simulink model "VehCtrlMdel240912_2018b"  (R2019b)
settings: Solver=FixedStepDiscrete  StartTime=0.0  StopTime=10.0  FixedStep=0.0005  RelTol=1e-3  EnableMultiTasking=on
values from neighbouring files (symbols this model uses):
  Ax_OffSet = 0.0    [VehCtrlMdelDictionary.sldd]
  Ay_OffSet = 0.0    [VehCtrlMdelDictionary.sldd]
  Caf = 460.0    [VehCtrlMdelDictionary.sldd]    (also in trqvparameter.m = 460)
  Car = 440.0    [VehCtrlMdelDictionary.sldd]    (also in trqvparameter.m = 440)
  dwf = 1.2    [VehCtrlMdelDictionary.sldd]    (also in trqvparameter.m)
  dwr = 1.2    [VehCtrlMdelDictionary.sldd]    (also in trqvparameter.m)
  h = 0.29    [VehCtrlMdelDictionary.sldd]    (also in trqvparameter.m)
  i1 = 11.4    [VehCtrlMdelDictionary.sldd]    (also in trqvparameter.m)
  i2 = 3.4    [VehCtrlMdelDictionary.sldd]    (also in trqvparameter.m)
  Iz = 105.0    [VehCtrlMdelDictionary.sldd]    (also in trqvparameter.m = 105)
  Kc = 1.0    [VehCtrlMdelDictionary.sldd]    (also in trqvparameter.m = 1)
  Ki = 1.0    [VehCtrlMdelDictionary.sldd]    (also in trqvparameter.m = 5)
  Ldwf = 1.2    [VehCtrlMdelDictionary.sldd]    (also in trqvparameter.m)
  Ldwr = 1.16    [VehCtrlMdelDictionary.sldd]    (also in trqvparameter.m)
  lf = 0.761    [VehCtrlMdelDictionary.sldd]    (also in trqvparameter.m)
  lr = 0.831    [VehCtrlMdelDictionary.sldd]    (also in trqvparameter.m)
  m = 340.0    [VehCtrlMdelDictionary.sldd]    (also in trqvparameter.m = 340)
  Offset_Angle = 0.0    [VehCtrlMdelDictionary.sldd]
  Qa = 0.1    [VehCtrlMdelDictionary.sldd]    (also in trqvparameter.m)
  Ra = 2.0    [VehCtrlMdelDictionary.sldd]    (also in trqvparameter.m = 2)
  Rt = 0.2    [VehCtrlMdelDictionary.sldd]    (also in trqvparameter.m)
  thr1 = 2.0    [VehCtrlMdelDictionary.sldd]    (also in trqvparameter.m = 2)
  thr2 = 0.5    [VehCtrlMdelDictionary.sldd]    (also in trqvparameter.m)
  thr3 = 0.8    [VehCtrlMdelDictionary.sldd]    (also in trqvparameter.m)
  thr4 = 0.5    [VehCtrlMdelDictionary.sldd]    (also in trqvparameter.m)
  thr5 = -0.5    [VehCtrlMdelDictionary.sldd]    (also in trqvparameter.m)
  TrqRquRate = 0.1    [VehCtrlMdelDictionary.sldd]    (also in trqvparameter.m)
  YawRate_OffSet = 0.0    [VehCtrlMdelDictionary.sldd]
undefined symbols (not defined in the file or in its folder): DiscIntNeverNeededParam, I_AN07_5V, I_AN08_5V, I_AN10_5V, I_SW01_L, I_SW02_L, I_SW03_L, O_SW12_HS1A, O_SW14_HS1A, PWM3
libraries: simulink x141, ec5744lib x77, canmsglib x18
(part 1 of 5)
settings Model: DataDictionary=VehCtrlMdelDictionary.sldd  EnableAccessToBaseWorkspace=off  Creator=YJR  LastModifiedBy=12045
settings DataIOCC: ReturnWorkspaceOutputs=off
settings OptimizationCC: DefaultParameterBehavior=Inlined  InlineInvariantSignals=on  EnhancedBackFolding=on  ExpressionFolding=off  PassReuseOutputArgsAs=Individual arguments  RollThreshold=65  StateBitsets=on  DataBitsets=on  ZeroExternalMemoryAtStartup=off  ZeroInternalMemoryAtStartup=off  EfficientFloat2IntCast=on  OptimizeBlockOrder=speed  DifferentSizesBufferReuse=on  EfficientTunableParamExpr=on
settings DebuggingCC: InheritedTsInSrcMsg=none  ParameterTunabilityLossMsg=error  ArithmeticOperatorsInVariantConditions=warning
settings HardwareCC: ProdBitPerPointer=32  ProdBitPerSizeT=32  ProdBitPerPtrDiffT=32  ProdLargestAtomicInteger=Long  ProdLargestAtomicFloat=Double  ProdEndianess=BigEndian  ProdWordSize=32  ProdHWDeviceType=Freescale MPC5500
settings SFSimCC: MATLABDynamicMemAlloc=off  CustomCodeUndefinedFunction=UseInterfaceOnly
settings RTWCC: Description=Target for EC5744  SystemTargetFile=ec5744.tlc  MakeCommand=make_rtw optimized_fixed_point=1  GenerateMakefile=off  TemplateMakefile=ec5744_lcc.tmf  PostCodeGenCommand=ec5744_pst_s2(buildInfo)  GenerateReport=on  IncludeHyperlinkInReport=on  LaunchReport=on  GenerateTraceInfo=on  GenerateTraceReport=on  GenerateTraceReportSl=on  GenerateTraceReportSf=on  GenerateTraceReportEml=on
settings CodeAppCC: ForceParamTrailComments=on  IgnoreCustomStorageClasses=off  OperatorAnnotations=on  SimulinkDataObjDesc=on  SFDataObjDesc=on  InsertBlockDesc=on
settings STFCustomTargetCC: TargetLangStandard=C99 (ISO)  MultiwordLength=256  ModelReferenceCompliant=off  IncludeMdlTerminateFcn=off  CombineOutputUpdateFcns=on  SuppressErrorStatus=on  ERTCustomFileBanners=on  SupportContinuousTime=off  SupportNonInlinedSFcns=off  RemoveResetFunc=on  MATLABClassNameForMDSCustomization=Simulink.SoftwareTarget.ERTCustomization  SystemTargetFile=ec5744.tlc
settings ERTTargetCC: TargetLangStandard=C99 (ISO)  ModelReferenceCompliant=off  ParMdlRefBuildCompliant=off  CompOptLevelCompliant=off  ConcurrentExecutionCompliant=off  IncludeMdlTerminateFcn=off  SuppressErrorStatus=on  ModelStepFunctionPrototypeControlCompliant=off  CPPClassGenCompliant=off  UseToolchainInfoCompliant=off  GenerateASAP2=on  InlinedParameterPlacement=NonHierarchical  ERTSrcFileBannerTemplate=ec5744_code_template.cgt  ERTHdrFileBannerTemplate=ec5744_code_template.cgt  ERTDataSrcFileTemplate=ec5744_code_template.cgt  ERTDataHdrFileTemplate=ec5744_code_template.cgt  ERTCustomFileTemplate=ec5744_file_process.tlc

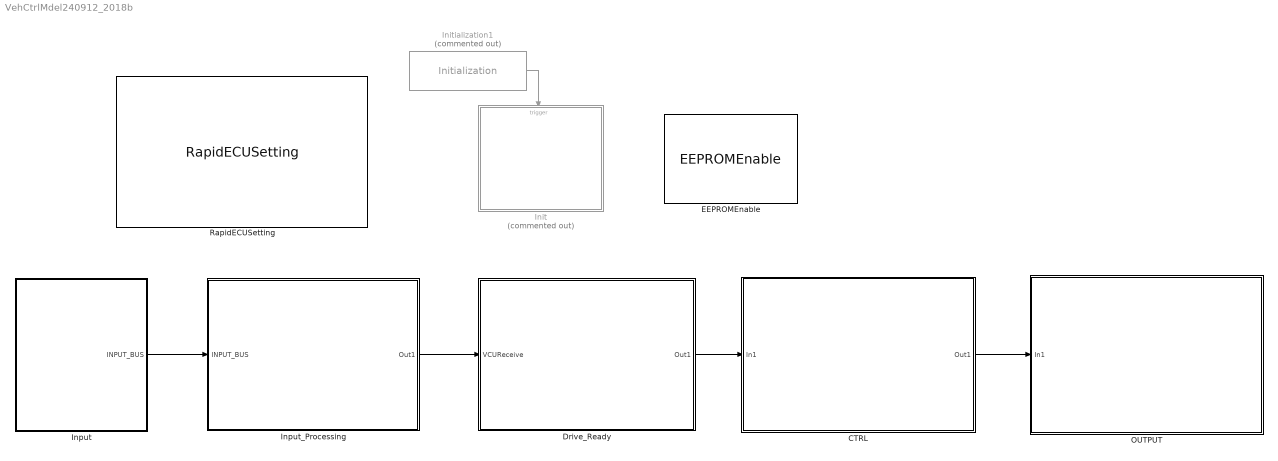
== system VehCtrlMdel240912_2018b ==
  CTRL : Subsystem
  Drive_Ready : Subsystem
  EEPROMEnable : ec5744lib/RapidECU_U3/09MemoryManagement/EEPROMEnable  eepromenable=on
      settings: SourceProductName=ECUCoder for MPC5744
  Init : Subsystem  Commented=on  TreatAsAtomicUnit=on
  Initialization1 : ec5744lib/RapidECU_U3/08MCUManagement/Initialization  Commented=on
      settings: SourceProductName=ECUCoder for MPC5744
  Input : Subsystem
  Input_Processing : Subsystem
  OUTPUT : Subsystem
  RapidECUSetting : ec5744lib/RapidECU_U3/RapidECUSetting
      link override CAN: apdf=9  bpdf=4  cpdf=4  acmt=Extended(29-bit ID)  bcmt=Standard(11-bit ID)  ccmt=Standard(11-bit ID)
      link override LIN: abrt=19200
      settings: SourceProductName=ECUCoder for MPC5744
  wires:
  Initialization1/1 -> Init/Trigger
  Input_Processing/1(Out1) -> Drive_Ready/1(VCUReceive)
  Input/1(INPUT_BUS) -> Input_Processing/1(INPUT_BUS)
  Drive_Ready/1(Out1) -> CTRL/1(In1)
  CTRL/1(Out1) -> OUTPUT/1(In1)

== system VehCtrlMdel240912_2018b/CTRL ==
  In1 : Inport
  10ms1 : simulink/Ports & Subsystems/Function-Call Generator  sample_time=0.01  numberOfIterations=1
  Bus Creator : BusCreator  Inputs=3
  Function-Call Generator : simulink/Ports & Subsystems/Function-Call Generator  sample_time=0.01  numberOfIterations=1
  MoTrqReq : Subsystem  TreatAsAtomicUnit=on
  PwrTrainTempPrtct : Subsystem
  Out1 : Outport  VectorParamsAs1DForOutWhenUnconnected=off
  wires:
  In1/1 -> MoTrqReq/2(In), [BUS], PwrTrainTempPrtct/1(In1)  "BUS"
  Function-Call Generator/1 -> PwrTrainTempPrtct/Trigger
  10ms1/1 -> MoTrqReq/Trigger
  PwrTrainTempPrtct/1(Out1) -> Bus Creator/1, [PwrTrainTempPrtct]  "WP_CTRL"
  [PwrTrainTempPrtct] -> MoTrqReq/1(In1)
  MoTrqReq/1(Motor_CtrlBus) -> Bus Creator/2  "Motor_CtrlBus"
  Bus Creator/1 -> Out1/1
  [BUS] -> Bus Creator/3

== system VehCtrlMdel240912_2018b/Drive_Ready ==
  VCUReceive : Inport
  10ms : simulink/Ports & Subsystems/Function-Call Generator  sample_time=0.01  numberOfIterations=1
  Bus Creator : BusCreator  Inputs=13
  Subsystem : Subsystem
  Out1 : Outport  VectorParamsAs1DForOutWhenUnconnected=off
  wires:
  VCUReceive/1 -> Subsystem/1(VCUReceive), Bus Creator/13  "VCUReceive"
  Subsystem/1(VehReady) -> Bus Creator/1
  Subsystem/2(BeeperStOut) -> Bus Creator/2
  Subsystem/3(VehStandby) -> Bus Creator/3
  Subsystem/4(AMKCANready) -> Bus Creator/4
  Subsystem/5(MCFL_DCOn_setpoints) -> Bus Creator/5
  Subsystem/6(MCFR_DCOn_setpoints) -> Bus Creator/6
  Subsystem/7(MCFL_DCEnable) -> Bus Creator/7
  Subsystem/8(MCFR_DCEnable) -> Bus Creator/8
  Subsystem/9(MCFL_InverterOn) -> Bus Creator/9
  Subsystem/10(MCFR_InverterOn) -> Bus Creator/10
  Subsystem/11(MC_DCOnError) -> Bus Creator/11
  10ms/1 -> Subsystem/Trigger
  Bus Creator/1 -> Out1/1
  Subsystem/12(errorReset) -> Bus Creator/12

== system VehCtrlMdel240912_2018b/Init ==
  function : TriggerPort  TriggerType=function-call  VariantControl=(inherit)
  AfterRunSwitch1 : ec5744lib/RapidECU_U3/05PowerManagement/AfterRunSwitch  sampletime=-1
      settings: SourceProductName=ECUCoder for MPC5744
  Constant : Constant  OutDataTypeStr=boolean
  Data Type Conversion : DataTypeConversion  OutDataTypeStr=boolean
  wires:
  Constant/1 -> Data Type Conversion/1
  Data Type Conversion/1 -> AfterRunSwitch1/1

== system VehCtrlMdel240912_2018b/Input ==
  10ms{,1..7} (8 alike) : simulink/Ports & Subsystems/Function-Call Generator  sample_time=0.01  numberOfIterations=1
  ABS_Receive : Subsystem  TreatAsAtomicUnit=on
  AMKMCU_Receive : Subsystem
  AccBrk_BUS : Subsystem
  BMS_Recive : Subsystem  TreatAsAtomicUnit=on
  Bus Creator : BusCreator  Inputs=8
  EMRAXMCU_RECIEVE : Subsystem  TreatAsAtomicUnit=on
  IMU_Recieve : Subsystem  TreatAsAtomicUnit=on
  StrSnis_Receive : Subsystem  TreatAsAtomicUnit=on
  key : Subsystem  TreatAsAtomicUnit=on
  INPUT_BUS : Outport  VectorParamsAs1DForOutWhenUnconnected=off
  wires:
  10ms2/1 -> IMU_Recieve/Trigger
  10ms/1 -> AccBrk_BUS/Trigger
  Bus Creator/1 -> INPUT_BUS/1  "VCUReceive"
  IMU_Recieve/1(IMU_BUS) -> Bus Creator/1
  AccBrk_BUS/1(AccBrk_BUS) -> Bus Creator/2  "AccBrk_BUS"
  AMKMCU_Receive/1(AMKMCUtoVCU_BUS) -> Bus Creator/3  "AMKMCUtoVCU_BUS"
  StrSnis_Receive/1(StrWhSnis_BUS) -> Bus Creator/4
  10ms4/1 -> StrSnis_Receive/Trigger
  10ms5/1 -> AMKMCU_Receive/Trigger
  BMS_Recive/1(BMS_BUS) -> Bus Creator/5
  10ms1/1 -> BMS_Recive/Trigger
  10ms3/1 -> ABS_Receive/Trigger
  ABS_Receive/1(ABS_BUS) -> Bus Creator/6
  10ms6/1 -> EMRAXMCU_RECIEVE/Trigger
  EMRAXMCU_RECIEVE/1(EMRAXMCU_Receive) -> Bus Creator/7  "EMRAXMCU_Receive"
  key/1(key) -> Bus Creator/8  "KEY"
  10ms7/1 -> key/Trigger

== system VehCtrlMdel240912_2018b/Input_Processing ==
  INPUT_BUS : Inport
  10ms : simulink/Ports & Subsystems/Function-Call Generator  sample_time=0.01  numberOfIterations=1
  10ms1 : simulink/Ports & Subsystems/Function-Call Generator  sample_time=0.01  numberOfIterations=1
  Bus Creator : BusCreator  Inputs=3
  Function-Call Subsystem : Subsystem  TreatAsAtomicUnit=on
  Subsystem : Subsystem
  Out1 : Outport  VectorParamsAs1DForOutWhenUnconnected=off
  wires:
  INPUT_BUS/1 -> Function-Call Subsystem/1(INPUT_BUS)
  10ms/1 -> Function-Call Subsystem/Trigger
  Function-Call Subsystem/1(Out1) -> [out], Bus Creator/1
  10ms1/1 -> Subsystem/Trigger
  Subsystem/1(VehVxEst_mps) -> Bus Creator/2  "VehVxEst_mps"
  Bus Creator/1 -> Out1/1
  [out] -> Subsystem/1(OutPutBus)  "out"
  Subsystem/2(Vxii_mps) -> Bus Creator/3  "Vxii_mps"

== system VehCtrlMdel240912_2018b/OUTPUT ==
  In1 : Inport
  10ms : simulink/Ports & Subsystems/Function-Call Generator  Commented=on  sample_time=0.01  numberOfIterations=1
  10ms{1..4,6} (5 alike) : simulink/Ports & Subsystems/Function-Call Generator  sample_time=0.01  numberOfIterations=1
  Beeper : Subsystem  TreatAsAtomicUnit=on
  Bus Selector : BusSelector  OutputSignals=Motor_CtrlBus,Motor_CtrlBus.TrqFL_cmd,BUS,Motor_CtrlBus.TrqFR_cmd,WP_CTRL.aWaterPumpON,WP_CTRL.LoadOfbWaterPump,BUS.BeeperStOut
  VCU2AMKMCUFL : Subsystem  TreatAsAtomicUnit=on
  VCU2AMKMCUFR : Subsystem  TreatAsAtomicUnit=on
  VCU2CLUSTER : Subsystem  Commented=on  TreatAsAtomicUnit=on
  VCU2EmraxMCU : Subsystem  TreatAsAtomicUnit=on
  WP_OUTPUT : Subsystem  TreatAsAtomicUnit=on
  wires:
  10ms3/1 -> VCU2EmraxMCU/Trigger
  In1/1 -> Bus Selector/1
  10ms2/1 -> VCU2AMKMCUFL/Trigger
  10ms4/1 -> VCU2AMKMCUFR/Trigger
  Bus Selector/1 -> VCU2EmraxMCU/1(In1)  "<Motor_CtrlBus>"
  Bus Selector/2 -> VCU2AMKMCUFL/1(MCFL_TargetTorque)  "<TrqFL_cmd>"
  Bus Selector/4 -> VCU2AMKMCUFR/2(In1)  "<TrqFR_cmd>"
  Bus Selector/3 -> VCU2AMKMCUFR/1(<BUS>), VCU2AMKMCUFL/2(In2)  "<BUS>"
  Bus Selector/5 -> WP_OUTPUT/1(aWaterPumpON)  "<aWaterPumpON>"
  10ms6/1 -> WP_OUTPUT/Trigger
  Bus Selector/7 -> Beeper/1(Beeper_state)  "<BeeperStOut>"
  10ms1/1 -> Beeper/Trigger
  Bus Selector/6 -> WP_OUTPUT/2(LoadOfbWaterPump)  "<LoadOfbWaterPump>"
  10ms/1 -> VCU2CLUSTER/Trigger

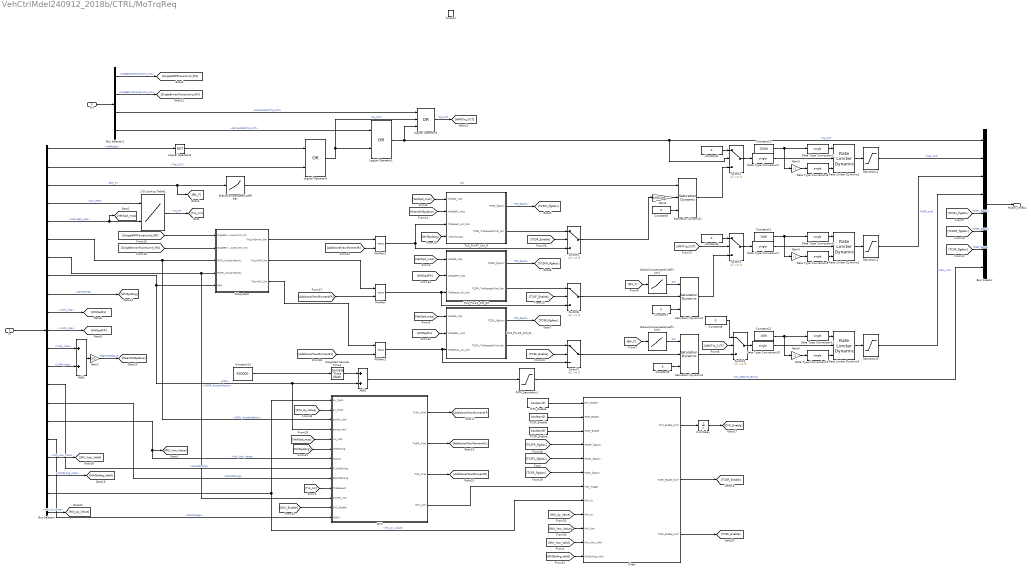
== system VehCtrlMdel240912_2018b/CTRL/MoTrqReq ==
  In1 : Inport
  In : Inport  Port=2
  function : TriggerPort  TriggerType=function-call  VariantControl=(inherit)
  2-D Lookup Table1 : Lookup_n-D  BreakpointsForDimension1=single([0 10 20 30 40 50 60 70 80 90 100])  BreakpointsForDimension2=single([5.40000009536743 10.8000001907349 16.2000007629395 21.6000003814697 27 32.4000015258789 37.7999992370605 43.2000007629395 48.5999984741211 54 59.4000015258789 64.8000030517578 70.1999969482422 75.5999984741211 81 86.4000015258789 91.8000030517578 97.1999969482422 102.599998474121 108])  BreakpointsForDimension1DataTypeStr=single  BreakpointsForDimension2DataTypeStr=single  Table=single([0 0 0 0 0 0 0 0 0 0 0 0 0 0 0 0 0 0 0 0;20 20 20 20 20 20 20 18 18 18 17 17 16 16 15 15 15 14 14 14;35 35 35 35 35 35 30 30 25 25 25 25 20 20 20 20 20 20 20 18;50 50 50 50 50 50 50 50 50 40 40 40 40 40 40 40 40 40 38 35;79 79 79 79 85 85 85 90 95 100 110 110 110 100 90 90 80 72 70 65;100 100 100 105 105 105 110 110 110 110 115 115 125 125 120 110 90 80 76 70;120 120 120 120 125 125 125 135 135 135 135 135 135 130 130 120 100 90 82 74;125 125 125 130 135 140 145 155 155 155 155 155 155 155 155 135 110 100 88 82;130 160 160 160 160 170 160 160 160 160 160 160 160 160 160 142 120 105 94 88;130 160 160 160 160 170 160 160 160 160 160 160 160 160 160 142 120 105 95 91;170 170 180 180 180 210 200 200 200 200 200 200 190 180 180 152 133 118 106 100])  InternalRulePriority=Speed  RndMeth=Simplest  InputSameDT=on
  Add1 : Sum
  Add2 : Sum
  BrakeCompensateCoefFront1 : Lookup_n-D  NumberOfTableDimensions=1  BreakpointsForDimension1=single([550,2000]);  Table=single([20,0]);  ExtrapMethod=Clip  InternalRulePriority=Speed  OutDataTypeStr=single  RndMeth=Simplest  InputSameDT=on
  BrakeCompensateCoefFront2 : Lookup_n-D  NumberOfTableDimensions=1  BreakpointsForDimension1=single([550,2000]);  Table=single([20,0]);  ExtrapMethod=Clip  InternalRulePriority=Speed  OutDataTypeStr=single  RndMeth=Simplest  InputSameDT=on
  BrakeCompensateCoefRear : Lookup_n-D  NumberOfTableDimensions=1  BreakpointsForDimension1=single([550,2000]);  Table=single([1000,0]);  ExtrapMethod=Clip  InternalRulePriority=Speed  OutDataTypeStr=single  RndMeth=Simplest  InputSameDT=on
  Bus Creator : BusCreator  Inputs=8
  Bus Selector : BusSelector  OutputSignals=VehReady,VCUReceive.signal1.AccBrkPedal_Processing.Trq_CUT,VCUReceive.signal1.AccBrkPedal_Processing.Brk_F,VCUReceive.signal1.AccBrkPedal_Processing.Acc_POS,VCUReceive.VehVxEst_mps,VCUReceive.signal1.BUS.AMKMCUtoVCU_BUS.FLAMKMCUtoVCU1.MCFL_ActualVelocity,VCUReceive.signal1.BUS.AMKMCUtoVCU_BUS.FRAMKMCUtoVCU1.MCFR_ActualVelocity,VCUReceive.signal1.BUS.EMRAXMCU_Receive.MCU_state.RPM,VCUReceive.signal1.SWAS_Processing.StrWhlAng,VCUReceive.Vxii_mps.VxFL_mps,VCUReceive.Vxii_mps.VxFR_mps,VCUReceive.Vxii_mps.VxRL_mps,VCUReceive.Vxii_mps.VxRR_mps,VCUReceive.signal1.SWAS_Processing.FLWhlStrAng,VCUReceive.signal1.SWAS_Processing.FRWhlStrAng,VCUReceive.signal1.IMU_Processing.IMU_Yaw_Value,VCUReceive.signal1.SWAS_Processing.StrWhlAngV,VCUReceive.signal1.IMU_Processing.IMU_Yaw_Valid,VCUReceive.signal1.SWAS_Processing.WhlStrAng_Valid,VCUReceive.signal1.IMU_Processing.IMU_Ax_Value,VCUReceive.signal1.IMU_Processing.IMU_Ay_Value
  Bus Selector1 : BusSelector  OutputSignals=SingleAMKPowerLimit_KW,SingleEmraxPowerLimit_KW,allAMKMotorTrq_CUT,EmraxMotorTrq_CUT
  Chart : Stateflow chart  TreatAsAtomicUnit=on
  Constant10 : Constant  Value=25000  OutDataTypeStr=single
  Constant11 : Constant  Value=1000  OutDataTypeStr=single
  Constant12 : Constant  Value=1000  OutDataTypeStr=single
  Constant13 : Constant  Value=420000  OutDataTypeStr=single
  Constant{4..9} (6 alike) : Constant  Value=0  OutDataTypeStr=single
  DTC_Enable : Constant  Value=boolean(0)
  DYC : Subsystem
  Data Type Conversion{1..2,6..12} (9 alike) : DataTypeConversion  OutDataTypeStr=single
  Gain2 : Gain  Gain=1/2
  Gain3 : Gain  Gain=-1
  Gain4 : Gain  Gain=-1
  Gain5 : Gain  Gain=-1
  Gain6 : Gain  Gain=1000/260
  Logical Operator1 : Logic  Operator=OR  AllPortsSameDT=off  OutDataTypeStr=boolean
  Logical Operator2 : Logic  Operator=NOT  AllPortsSameDT=off  OutDataTypeStr=boolean
  Logical Operator3 : Logic  Operator=OR  AllPortsSameDT=off  OutDataTypeStr=boolean
  Logical Operator4 : Logic  Operator=OR  Inputs=3  AllPortsSameDT=off  OutDataTypeStr=boolean
  MinMax : MinMax  Inputs=2
  MinMax1 : MinMax  Inputs=2
  MinMax2 : MinMax  Inputs=2
  RPM_Saturation1 : Saturate  UpperLimit=5000  LowerLimit=-50
  Rate Limiter Dynamic1 : simulink/Discontinuities/Rate Limiter Dynamic
      settings: SourceProductName=Simulink
  Rate Limiter Dynamic2 : simulink/Discontinuities/Rate Limiter Dynamic
      settings: SourceProductName=Simulink
  Rate Limiter Dynamic3 : simulink/Discontinuities/Rate Limiter Dynamic
      settings: SourceProductName=Simulink
  Saturation Dynamic1 : simulink/Discontinuities/Saturation Dynamic  OutMin=[]  OutMax=[]  OutDataTypeStr=single  OutputDataTypeScalingMode=single  OutDataType=fixdt(1, 16)  OutScaling=2^-10  DoSatur=off
  Saturation Dynamic2 : simulink/Discontinuities/Saturation Dynamic  OutMin=[]  OutMax=[]  OutDataTypeStr=single  OutputDataTypeScalingMode=single  OutDataType=fixdt(1, 16)  OutScaling=2^-10  DoSatur=off
  Saturation Dynamic3 : simulink/Discontinuities/Saturation Dynamic  OutMin=[]  OutMax=[]  OutDataTypeStr=single  OutputDataTypeScalingMode=single  OutDataType=fixdt(1, 16)  OutScaling=2^-10  DoSatur=off
  Saturation1 : Saturate  UpperLimit=1000  LowerLimit=0
  Saturation2 : Saturate  UpperLimit=20  LowerLimit=0
  Saturation3 : Saturate  UpperLimit=20  LowerLimit=0
  Subsystem : Subsystem
  Switch{2..7} (6 alike) : Switch  Criteria=u2 ~= 0
  TCSF_Enable : Constant  Value=boolean(0)  OutDataTypeStr=boolean
  TCSR_Enable : Constant  Value=boolean(0)  OutDataTypeStr=boolean
  TCS_PI+FF_Ctrl_FL : Subsystem
  TCS_PI+FF_Ctrl_FR : Subsystem
  TCS_PI+FF_Ctrl_R : Subsystem
  Unit Delay : UnitDelay  SampleTime=-1  HasFrameUpgradeWarning=on
  Weighted Sample Time1 : SampleTimeMath  TsampMathOp=*
  Motor_CtrlBus : Outport  VectorParamsAs1DForOutWhenUnconnected=off
  wires:
  In/1 -> Bus Selector/1
  Bus Creator/1 -> Motor_CtrlBus/1
  Bus Selector/4 -> 2-D Lookup Table1/1  "<Acc_POS>"
  Bus Selector/5 -> [VehSpd_mps], 2-D Lookup Table1/2  "<VehVxEst_mps>"
  Bus Selector/1 -> Logical Operator2/1  "<VehReady>"
  Bus Selector/2 -> Logical Operator3/2  "<Trq_CUT>"
  Logical Operator2/1 -> Logical Operator3/1
  Logical Operator1/1 -> Switch2/2, Bus Creator/1, Logical Operator4/3  "Trq_CUT"
  Constant4/1 -> Switch2/1
  Bus Selector/3 -> [Brk_F], BrakeCompensateCoefRear/1  "<Brk_F>"
  Saturation Dynamic1/1 -> Switch2/3
  Switch2/1 -> Data Type Conversion1/1
  BrakeCompensateCoefRear/1 -> Saturation Dynamic1/1  "pct"
  2-D Lookup Table1/1 -> [Trq_nm]  "Trq_nm"
  Bus Selector/6 -> DYC/3(amkFL_rpm), Subsystem/3(MCFL_ActualVelocity)  "<MCFL_ActualVelocity>"
  Bus Selector/7 -> DYC/11(amkFR_rpm), Subsystem/4(MCFR_ActualVelocity)  "<MCFR_ActualVelocity>"
  Bus Selector/8 -> Subsystem/5(RPM), DYC/4(emrax_rpm), Add2/2  "<RPM>"
  Subsystem/1(TrqLimEmrax_Nm) -> MinMax2/1
  Switch5/1 -> Gain6/1
  Constant5/1 -> Saturation Dynamic1/3
  [VehSpd_mps] -> TCS_PI+FF_Ctrl_R/1(VehSpd_mps)
  [VehSpd_mps] -> TCS_PI+FF_Ctrl_FR/1(VehSpd_mps)
  [VehSpd_mps] -> TCS_PI+FF_Ctrl_FL/1(VehSpd_mps)
  Bus Selector/9 -> [WhlSpdAng]  "<StrWhlAng>"
  Constant6/1 -> Switch3/1
  [AMKTrq_CUT] -> Switch3/2
  TCS_PI+FF_Ctrl_FR/2(TCSFR_TrqRequestFinal_Nm) -> Switch6/1
  Constant7/1 -> Saturation Dynamic2/3
  Saturation Dynamic2/1 -> Switch3/3
  [Brk_F] -> BrakeCompensateCoefFront2/1
  BrakeCompensateCoefFront2/1 -> Saturation Dynamic3/1  "pct"
  TCS_PI+FF_Ctrl_FL/2(TCSFL_TrqRequestFinal_Nm) -> Switch7/1
  Saturation Dynamic3/1 -> Switch4/3
  [AMKTrq_CUT] -> Switch4/2
  Constant8/1 -> Switch4/1
  TCS_PI+FF_Ctrl_R/1(TCSR_flgActv) -> [TCSFL_flgActv]  "TCS_flgActv"
  [TCSFL_flgActv] -> Bus Creator/5  "TCSFL_flgActv"
  TCS_PI+FF_Ctrl_FR/1(TCSFR_flgActv) -> [TCSFR_flgActv]  "TCS_flgActv"
  [TCSFR_flgActv] -> Bus Creator/6  "TCSFR_flgActv"
  TCS_PI+FF_Ctrl_FL/1(TCSFL_flgActv) -> [TCSR_flgActv]  "TCS_flgActv"
  [TCSR_flgActv] -> Bus Creator/7  "TCSR_flgActv"
  Constant9/1 -> Saturation Dynamic3/3
  Bus Selector/12 -> Add1/1  "<VxRL_mps>"
  Bus Selector/13 -> Add1/2  "<VxRR_mps>"
  Bus Selector/11 -> [WhlSpdFR]  "<VxFR_mps>"
  Bus Selector/10 -> [WhlSpdFL]  "<VxFL_mps>"
  Add1/1 -> Gain2/1
  Gain2/1 -> [RearWhlSpdAve]  "RearWhlSpdAve"
  [WhlSpdFL] -> TCS_PI+FF_Ctrl_FL/2(VehSpdFL_mps)
  [RearWhlSpdAve] -> TCS_PI+FF_Ctrl_R/2(VehSpdFL_mps)
  [WhlSpdFR] -> TCS_PI+FF_Ctrl_FR/2(VehSpdFR_mps)
  Switch3/1 -> Data Type Conversion7/1
  Switch4/1 -> Data Type Conversion10/1
  Constant10/1 -> Gain3/1, Data Type Conversion2/1
  Gain3/1 -> Data Type Conversion6/1
  Data Type Conversion2/1 -> Rate Limiter Dynamic1/1
  Data Type Conversion1/1 -> Rate Limiter Dynamic1/2
  Data Type Conversion6/1 -> Rate Limiter Dynamic1/3
  Rate Limiter Dynamic1/1 -> Saturation1/1
  Rate Limiter Dynamic2/1 -> Saturation2/1
  Data Type Conversion9/1 -> Rate Limiter Dynamic2/3
  Data Type Conversion7/1 -> Rate Limiter Dynamic2/2
  Data Type Conversion8/1 -> Rate Limiter Dynamic2/1
  Gain4/1 -> Data Type Conversion9/1
  Constant11/1 -> Data Type Conversion8/1, Gain4/1
  Constant12/1 -> Gain5/1, Data Type Conversion11/1
  Gain5/1 -> Data Type Conversion12/1
  Data Type Conversion11/1 -> Rate Limiter Dynamic3/1
  Data Type Conversion10/1 -> Rate Limiter Dynamic3/2
  Data Type Conversion12/1 -> Rate Limiter Dynamic3/3
  Rate Limiter Dynamic3/1 -> Saturation3/1
  Saturation3/1 -> Bus Creator/4  "TrqFL_cmd"
  Gain6/1 -> Saturation Dynamic1/2
  Weighted Sample Time1/1 -> Add2/1
  Constant13/1 -> Weighted Sample Time1/1
  RPM_Saturation1/1 -> Bus Creator/8  "VCU_SpdCmd_Emrax"
  Add2/1 -> RPM_Saturation1/1
  MinMax2/1 -> TCS_PI+FF_Ctrl_R/3(TrqRequst_Act_Nm), Switch5/3
  MinMax/1 -> Switch6/3, TCS_PI+FF_Ctrl_FR/3(TrqRequst_Act_Nm)
  MinMax1/1 -> Switch7/3, TCS_PI+FF_Ctrl_FL/3(TrqRequst_Act_Nm)
  TCS_PI+FF_Ctrl_R/2(TCSR_TrqRequestFinal_Nm) -> Switch5/1
  [TCSR_Enable] -> Switch5/2
  Switch6/1 -> Saturation Dynamic2/2
  [TCSF_Enable] -> Switch6/2
  Switch7/1 -> Saturation Dynamic3/2
  [TCSF_Enable] -> Switch7/2
  Saturation1/1 -> Bus Creator/2  "TrqR_cmd"
  Saturation2/1 -> Bus Creator/3  "TrqFR_cmd"
  BrakeCompensateCoefFront1/1 -> Saturation Dynamic2/1  "pct"
  [Brk_F] -> BrakeCompensateCoefFront1/1
  Subsystem/2(TrqLimFR_Nm) -> MinMax/1
  Subsystem/3(TrqLimFL_Nm) -> MinMax1/1
  In1/1 -> Bus Selector1/1
  Bus Selector1/4 -> Logical Operator1/1  "<EmraxMotorTrq_CUT>"
  Bus Selector1/3 -> Logical Operator4/1  "<allAMKMotorTrq_CUT>"
  Bus Selector1/1 -> [SingleAMKPowerLimit_KW]  "<SingleAMKPowerLimit_KW>"
  Bus Selector1/2 -> [SingleEmraxPowerLimit_KW]  "<SingleEmraxPowerLimit_KW>"
  [SingleAMKPowerLimit_KW] -> Subsystem/1(SingleAMKPowerLimit_KW)
  [SingleEmraxPowerLimit_KW] -> Subsystem/2(SingleEmraxPowerLimit_KW)
  DYC/1(TrqFL_Final) -> [AdditionalYawMomentFR]
  DYC/2(TrqFR_Final) -> [AdditionalYawMomentFL]
  [AdditionalYawMomentFR] -> MinMax/2
  [AdditionalYawMomentFL] -> MinMax1/2
  [VehSpd_mps] -> DYC/5(Vx_mps)
  Bus Selector/14 -> DYC/8(FLWhlStrAng)  "<FLWhlStrAng>"
  Bus Selector/15 -> DYC/9(FRWhlStrAng)  "<FRWhlStrAng>"
  Bus Selector/16 -> DYC/7(Wactul), [IMU_Yaw_Value]  "<IMU_Yaw_Value>"
  Bus Selector/17 -> DYC/13(WSAV)  "<StrWhlAngV>"
  [WhlSpdAng] -> TCS_PI+FF_Ctrl_R/4(<StrWhlAng>)
  DTC_Enable/1 -> Chart/1(DYC_Enable)
  TCSF_Enable/1 -> Chart/2(TCSF_Enable)
  TCSR_Enable/1 -> Chart/3(TCSR_Enable)
  Logical Operator3/1 -> Logical Operator4/2, Logical Operator1/2  "Trq_CUT"
  Logical Operator4/1 -> [AMKTrq_CUT]  "Trq_CUT"
  Bus Selector/18 -> [IMU_Yaw_Valid]  "<IMU_Yaw_Valid>"
  Bus Selector/19 -> [WhlStrAng_Valid]  "<WhlStrAng_Valid>"
  DYC/4(DYC_Actv) -> Chart/7(TVD_Trigger)
  [TCSFR_flgActv] -> Chart/4(TCSFR_flgActv)
  [TCSFL_flgActv] -> Chart/5(TCSFL_flgActv)
  [TCSR_flgActv] -> Chart/6(TCSR_flgActv)
  Chart/1(DYC_Enable_OUT) -> Unit Delay/1
  Chart/2(TCSR_Enable_OUT) -> [TCSR_Enable]
  Chart/3(TCSF_Enable_OUT) -> [TCSF_Enable]
  Bus Selector/20 -> DYC/1(ax_mpss), Chart/8(IMU_Ax)  "<IMU_Ax_Value>"
  [IMU_Yaw_Value] -> Chart/10(IMU_Yaw)
  [WhlSpdAng] -> DYC/6(WhlStrAng)
  DYC/3(TrqR_Final) -> [AdditionalYawMomentR]
  [DYC_Enable] -> DYC/12(DYC_Enable)
  [AdditionalYawMomentR] -> MinMax2/2
  Unit Delay/1 -> [DYC_Enable]
  [IMU_Yaw_Valid] -> Chart/11(IMU_Yaw_Valid)
  [WhlStrAng_Valid] -> Chart/12(WhlStrAng_Valid)
  [IMU_Ay_Value] -> Chart/9(IMU_Ay)
  Bus Selector/21 -> [IMU_Ay_Value]  "<IMU_Ay_Value>"
  [IMU_Ay_Value] -> DYC/2(ay_mpss)
  [Trq_nm] -> DYC/10(TrqRequest)

== system VehCtrlMdel240912_2018b/CTRL/PwrTrainTempPrtct ==
  In1 : Inport
  function : TriggerPort  TriggerType=function-call  VariantControl=(inherit)
  2-D Lookup Table1 : Lookup_n-D  NumberOfTableDimensions=1  BreakpointsForDimension1=[35,40,41,42,43,44,45,50]  BreakpointsForDimension2=[1:3]  Table=[0,0,0.2,0.4,0.6,0.8,1,1]  InternalRulePriority=Speed  RndMeth=Simplest  InputSameDT=on
  2-D Lookup Table2 : Lookup_n-D  NumberOfTableDimensions=1  BreakpointsForDimension1=[0;25;30;35;37;40;50]  BreakpointsForDimension2=[1:3]  Table=[0;0;20;40;70;100;100]  InternalRulePriority=Speed  RndMeth=Simplest  InputSameDT=on
  2-D Lookup Table3 : Lookup_n-D  NumberOfTableDimensions=1  BreakpointsForDimension1=[35,40,41,42,43,44,45,50]  BreakpointsForDimension2=[1:3]  Table=[0,0,0.2,0.4,0.6,0.8,1,1]  InternalRulePriority=Speed  RndMeth=Simplest  InputSameDT=on
  AND : Logic  AllPortsSameDT=off  OutDataTypeStr=boolean
  AND1 : Logic  AllPortsSameDT=off  OutDataTypeStr=boolean
  Bus Selector : BusSelector  OutputSignals=VCUReceive.signal1.BUS.AMKMCUtoVCU_BUS.FLAMKMCUtoVCU3.MCFL_TempInverter,VCUReceive.signal1.BUS.AMKMCUtoVCU_BUS.FRAMKMCUtoVCU3.MCFR_TempInverter,VCUReceive.signal1.BUS.EMRAXMCU_Receive.MCU_pwr.MCU_temp,VCUReceive.signal1.BUS.EMRAXMCU_Receive.MCU_pwr.motor_temp
  Bus Creator : BusCreator  Inputs=6
  Cast To Boolean : DataTypeConversion  OutDataTypeStr=boolean
  Cast To Boolean1 : DataTypeConversion  OutDataTypeStr=boolean
  Cast To Boolean2 : DataTypeConversion  OutDataTypeStr=boolean
  Cast To Single : DataTypeConversion  OutDataTypeStr=single
  Compare To Constant : simulink/Logic and Bit Operations/Compare To Constant  relop=>  const=40  OutDataTypeStr=boolean
  Compare To Constant1 : simulink/Logic and Bit Operations/Compare To Constant  relop=>  const=45  OutDataTypeStr=boolean
  Compare To Constant2 : simulink/Logic and Bit Operations/Compare To Constant  relop=>  const=45  OutDataTypeStr=boolean
  Compare To Constant3 : simulink/Logic and Bit Operations/Compare To Constant  relop=>  const=50  OutDataTypeStr=boolean
  Compare To Constant4 : simulink/Logic and Bit Operations/Compare To Constant  relop=>  const=35  OutDataTypeStr=boolean
  Constant : Constant  Value=single(0)
  Constant1 : Constant  Value=single(0)
  Constant2 : Constant  Value=single(0.11)
  Constant3 : Constant  Value=single(0.11)
  Gain : Gain  Gain=10
  Max : MinMax  Function=max  Inputs=2
  Max1 : MinMax  Function=max  Inputs=2
  NOT : Logic  Operator=NOT  AllPortsSameDT=off  OutDataTypeStr=boolean
  NOT1 : Logic  Operator=NOT  AllPortsSameDT=off  OutDataTypeStr=boolean
  Switch : Switch  Criteria=u2 ~= 0
  Switch1 : Switch  Criteria=u2 ~= 0
  Timer1 : Stateflow chart  TreatAsAtomicUnit=on
  Timer2 : Stateflow chart  TreatAsAtomicUnit=on
  Out1 : Outport  VectorParamsAs1DForOutWhenUnconnected=off
  wires:
  Compare To Constant1/1 -> Cast To Boolean/1, NOT/1
  Max/1 -> Compare To Constant4/1, 2-D Lookup Table1/1, Compare To Constant/1, Compare To Constant1/1
  Compare To Constant/1 -> AND/1
  Constant/1 -> Switch/3
  NOT/1 -> AND/2
  AND/1 -> Switch/2
  Switch/1 -> Bus Creator/1  "SingleAMKPowerLimit_KW"
  Bus Selector/2 -> Max/2  "<MCFR_TempInverter>"
  2-D Lookup Table1/1 -> Switch/1
  Timer1/1(Exit) -> Bus Creator/2  "allAMKMotorTrq_CUT"
  Compare To Constant4/1 -> Cast To Boolean2/1  "aWaterPumpON"
  Timer2/1(Exit) -> Bus Creator/5  "EmraxMotorTrq_CUT"
  2-D Lookup Table3/1 -> Switch1/1
  Switch1/1 -> Bus Creator/4  "SingleEmraxPowerLimit_KW"
  AND1/1 -> Switch1/2
  NOT1/1 -> AND1/2
  Constant1/1 -> Switch1/3
  Compare To Constant2/1 -> AND1/1
  Bus Selector/3 -> Max1/1, Compare To Constant3/1, Compare To Constant2/1  "<MCU_temp>"
  Compare To Constant3/1 -> NOT1/1, Cast To Boolean1/1
  Bus Selector/4 -> Max1/2  "<motor_temp>"
  2-D Lookup Table2/1 -> Cast To Single/1  "LoadOfbWaterPump"
  In1/1 -> Bus Selector/1
  Bus Selector/1 -> Max/1  "<MCFL_TempInverter>"
  Max1/1 -> [MAXEmraxTemp], 2-D Lookup Table2/1
  [MAXEmraxTemp] -> 2-D Lookup Table3/1
  Bus Creator/1 -> Out1/1
  Cast To Boolean2/1 -> Bus Creator/3  "aWaterPumpON"
  Gain/1 -> Bus Creator/6  "LoadOfbWaterPump"
  Cast To Single/1 -> Gain/1
  Constant2/1 -> Timer1/2(CountTime)
  Cast To Boolean/1 -> Timer1/1(Trigger)
  Constant3/1 -> Timer2/2(CountTime)
  Cast To Boolean1/1 -> Timer2/1(Trigger)

== system VehCtrlMdel240912_2018b/Drive_Ready/Subsystem ==
  VCUReceive : Inport
  function : TriggerPort  TriggerType=function-call  VariantControl=Variant
  Bus Selector : BusSelector  OutputSignals=signal1.AccBrkPedal_Processing.Brk_F,signal1.BUS.KEY.ignition,signal1.AccBrkPedal_Processing.Acc_POS,signal1.BUS.EMRAXMCU_Receive.MCU_state.controller_ready,signal1.BUS.AMKMCUtoVCU_BUS.FLAMKMCUtoVCU1.MCFL_bSystemReady,signal1.BUS.AMKMCUtoVCU_BUS.FRAMKMCUtoVCU1.MCFR_bSystemReady,signal1.BUS.AMKMCUtoVCU_BUS.FLAMKMCUtoVCU1.MCFL_bDCOn,signal1.BUS.AMKMCUtoVCU_BUS.FRAMKMCUtoVCU1.MCFR_bDCOn,signal1.BUS.KEY.AMKCLDCON,signal1.BUS.KEY.HVCUTOFF
  Cast To Boolean : DataTypeConversion  OutDataTypeStr=boolean
  Chart2 : Stateflow chart  TreatAsAtomicUnit=on
  Compare To Constant : simulink/Logic and Bit Operations/Compare To Constant  relop=>=  const=450  OutDataTypeStr=boolean
  Compare To Constant1 : simulink/Logic and Bit Operations/Compare To Constant  relop=<=  const=50  OutDataTypeStr=boolean
  VehReady : Outport
  BeeperStOut : Outport  Port=2
  VehStandby : Outport  Port=3
  AMKCANready : Outport  Port=4
  MCFL_DCOn_setpoints : Outport  Port=5
  MCFR_DCOn_setpoints : Outport  Port=6
  MCFL_DCEnable : Outport  Port=7
  MCFR_DCEnable : Outport  Port=8
  MCFL_InverterOn : Outport  Port=9
  MCFR_InverterOn : Outport  Port=10
  MC_DCOnError : Outport  Port=11
  errorReset : Outport  Port=12
  wires:
  Bus Selector/10 -> Chart2/12(HVCutOFF)  "<HVCUTOFF>"
  Chart2/1(VehReady) -> VehReady/1
  Chart2/4(AMKCANready) -> AMKCANready/1
  Chart2/2(BeeperStOut) -> BeeperStOut/1
  Bus Selector/9 -> Chart2/11(SWAMKDCOn)  "<AMKCLDCON>"
  Chart2/5(MCFL_DCOn_setpoints) -> MCFL_DCOn_setpoints/1
  Compare To Constant1/1 -> Chart2/3(ACC_Release)  "ACC_Release"
  Chart2/7(MCFR_DCEnable) -> MCFR_DCEnable/1
  Chart2/8(MCFR_InverterOn) -> MCFR_InverterOn/1
  Compare To Constant/1 -> Chart2/1(Brk)  "Brk"
  Chart2/9(MC_DCOnError) -> MC_DCOnError/1
  Chart2/11(MCFL_DCEnable) -> MCFL_DCEnable/1
  Chart2/3(VehStandby) -> VehStandby/1
  Bus Selector/6 -> Chart2/6(bMCUReady), Chart2/10(MCFR_SYSREADY)  "<MCFR_bSystemReady>"
  Chart2/6(MCFR_DCOn_setpoints) -> MCFR_DCOn_setpoints/1
  Cast To Boolean/1 -> Chart2/2(KeyPressed)  "KeyPressed"
  Bus Selector/7 -> Chart2/8(MCFLDCOncheck)  "<MCFL_bDCOn>"
  Chart2/10(MCFL_InverterOn) -> MCFL_InverterOn/1
  VCUReceive/1 -> Bus Selector/1
  Bus Selector/1 -> Compare To Constant/1  "<Brk_F>"
  Bus Selector/2 -> Cast To Boolean/1  "<ignition>"
  Bus Selector/3 -> Compare To Constant1/1  "<Acc_POS>"
  Bus Selector/4 -> Chart2/4(cMCUReady)  "<controller_ready>"
  Bus Selector/5 -> Chart2/5(aMCUReady), Chart2/9(MCFL_SYSREADY)  "<MCFL_bSystemReady>"
  Bus Selector/8 -> Chart2/7(MCFRDCOncheck)  "<MCFR_bDCOn>"
  Chart2/12(errorReset) -> errorReset/1

== system VehCtrlMdel240912_2018b/Input/ABS_Receive ==
  function : TriggerPort  TriggerType=function-call  VariantControl=Variant
  ABS_BUS_state : Subsystem  TreatAsAtomicUnit=on
  CANReceive3 : ec5744lib/RapidECU_U3/04CANCommunication/CANReceive  canmodule=0  canbuffer=16  canmessageid=1698  canmessagetype=Standard(11-bit ID)  datalength=8  sampletime=-1
      settings: SourceProductName=ECUCoder for MPC5744
  Terminator3 : Terminator
  ABS_BUS : Outport  VectorParamsAs1DForOutWhenUnconnected=off
  wires:
  CANReceive3/3 -> ABS_BUS_state/2(ID)
  CANReceive3/4 -> ABS_BUS_state/3(Msg)
  CANReceive3/1 -> ABS_BUS_state/Trigger
  ABS_BUS_state/1(ABS_BUS) -> ABS_BUS/1  "ABS_BUS"
  CANReceive3/5 -> Terminator3/1
  CANReceive3/2 -> ABS_BUS_state/1(CANOK)

== system VehCtrlMdel240912_2018b/Input/AMKMCU_Receive ==
  function : TriggerPort  TriggerType=function-call  VariantControl=Variant
  Bus Creator : BusCreator  Inputs=6
  FLAMKMCU : Subsystem
  FRAMKMCU : Subsystem
  AMKMCUtoVCU_BUS : Outport  VectorParamsAs1DForOutWhenUnconnected=off
  wires:
  Bus Creator/1 -> AMKMCUtoVCU_BUS/1
  FLAMKMCU/1(FLAMKMCUtoVCU1) -> Bus Creator/1
  FLAMKMCU/2(FLAMKMCUtoVCU2) -> Bus Creator/2  "FLAMKMCUtoVCU2"
  FLAMKMCU/3(FLAMKMCUtoVCU3) -> Bus Creator/3
  FRAMKMCU/1(FRAMKMCUtoVCU1) -> Bus Creator/4
  FRAMKMCU/2(FRAMKMCUtoVCU2) -> Bus Creator/5
  FRAMKMCU/3(FRAMKMCUtoVCU3) -> Bus Creator/6

== system VehCtrlMdel240912_2018b/Input/AccBrk_BUS ==
  function : TriggerPort  TriggerType=function-call  VariantControl=Variant
  Acc1 : ec5744lib/RapidECU_U3/01BasicInput/AnalogInput  channel=56:I_AN10_5V  sampletime=-1
      settings: SourceProductName=ECUCoder for MPC5744
  Acc2 : ec5744lib/RapidECU_U3/01BasicInput/AnalogInput  channel=53:I_AN07_5V  sampletime=-1
      settings: SourceProductName=ECUCoder for MPC5744
  Brk1 : ec5744lib/RapidECU_U3/01BasicInput/AnalogInput  channel=54:I_AN08_5V  sampletime=-1
      settings: SourceProductName=ECUCoder for MPC5744
  Bus Creator : BusCreator  Inputs=3
  AccBrk_BUS : Outport  VectorParamsAs1DForOutWhenUnconnected=off
  wires:
  Brk1/1 -> Bus Creator/2  "Brk1"
  Acc1/1 -> Bus Creator/1  "Acc1"
  Bus Creator/1 -> AccBrk_BUS/1
  Acc2/1 -> Bus Creator/3  "Acc2"

== system VehCtrlMdel240912_2018b/Input/BMS_Recive ==
  function : TriggerPort  TriggerType=function-call  VariantControl=Variant
  ABS_BUS_state : Subsystem  TreatAsAtomicUnit=on
  CANReceive3 : ec5744lib/RapidECU_U3/04CANCommunication/CANReceive  canmodule=0  canbuffer=16  canmessageid=1698  canmessagetype=Standard(11-bit ID)  datalength=8  sampletime=-1
      settings: SourceProductName=ECUCoder for MPC5744
  Terminator3 : Terminator
  BMS_BUS : Outport  VectorParamsAs1DForOutWhenUnconnected=off
  wires:
  ABS_BUS_state/1(BMS_BUS) -> BMS_BUS/1  "BMS_BUS"
  CANReceive3/3 -> ABS_BUS_state/2(ID)
  CANReceive3/1 -> ABS_BUS_state/Trigger
  CANReceive3/2 -> ABS_BUS_state/1(CANOK)
  CANReceive3/5 -> Terminator3/1
  CANReceive3/4 -> ABS_BUS_state/3(Msg)

== system VehCtrlMdel240912_2018b/Input/EMRAXMCU_RECIEVE ==
  function : TriggerPort  TriggerType=function-call  VariantControl=(inherit)
  Bus Creator2 : BusCreator  Inputs=2
  CANReceive1 : ec5744lib/RapidECU_U3/04CANCommunication/CANReceive  canmodule=0  canbuffer=1  canmessageid=218089455  canmessagetype=Extended(29-bit ID)  datalength=8  sampletime=-1
      settings: SourceProductName=ECUCoder for MPC5744
  CANReceive3 : ec5744lib/RapidECU_U3/04CANCommunication/CANReceive  canmodule=0  canbuffer=0  canmessageid=218089199  canmessagetype=Extended(29-bit ID)  datalength=8  sampletime=-1
      settings: SourceProductName=ECUCoder for MPC5744
  MCU_pwr : Subsystem  TreatAsAtomicUnit=on
  MCU_state : Subsystem  TreatAsAtomicUnit=on
  Terminator1 : Terminator
  Terminator3 : Terminator
  EMRAXMCU_Receive : Outport
  wires:
  CANReceive1/3 -> MCU_pwr/2(ID)
  CANReceive1/4 -> MCU_pwr/3(Msg)
  CANReceive1/2 -> MCU_pwr/1(CANOK)
  CANReceive3/1 -> MCU_state/Trigger
  CANReceive1/1 -> MCU_pwr/Trigger
  MCU_pwr/1(MCU_pwr) -> Bus Creator2/2  "MCU_pwr"
  CANReceive3/2 -> MCU_state/1(CANOK)
  CANReceive3/5 -> Terminator3/1
  CANReceive1/5 -> Terminator1/1
  MCU_state/1(Out1) -> Bus Creator2/1  "MCU_state"
  CANReceive3/3 -> MCU_state/2(ID)
  CANReceive3/4 -> MCU_state/3(Msg)
  Bus Creator2/1 -> EMRAXMCU_Receive/1

== system VehCtrlMdel240912_2018b/Input/IMU_Recieve ==
  function : TriggerPort  TriggerType=function-call  VariantControl=Variant
  CANReceive3 : ec5744lib/RapidECU_U3/04CANCommunication/CANReceive  canmodule=0  canbuffer=0  canmessageid=513  canmessagetype=Standard(11-bit ID)  datalength=8  sampletime=-1
      settings: SourceProductName=ECUCoder for MPC5744
  IMU_state : Subsystem  TreatAsAtomicUnit=on
  Terminator3 : Terminator
  IMU_BUS : Outport  VectorParamsAs1DForOutWhenUnconnected=off
  wires:
  CANReceive3/3 -> IMU_state/2(ID)
  CANReceive3/1 -> IMU_state/Trigger
  IMU_state/1(IMU_BUS) -> IMU_BUS/1  "IMU"
  CANReceive3/2 -> IMU_state/1(CANOK)
  CANReceive3/5 -> Terminator3/1
  CANReceive3/4 -> IMU_state/3(Msg)

== system VehCtrlMdel240912_2018b/Input/StrSnis_Receive ==
  function : TriggerPort  TriggerType=function-call  VariantControl=Variant
  CANReceive3 : ec5744lib/RapidECU_U3/04CANCommunication/CANReceive  canmodule=0  canbuffer=7  canmessageid=330  canmessagetype=Standard(11-bit ID)  datalength=8  sampletime=-1
      settings: SourceProductName=ECUCoder for MPC5744
  StrWhSnis_state : Subsystem  TreatAsAtomicUnit=on
  Terminator3 : Terminator
  StrWhSnis_BUS : Outport  VectorParamsAs1DForOutWhenUnconnected=off
  wires:
  CANReceive3/2 -> StrWhSnis_state/1(CANOK)
  CANReceive3/5 -> Terminator3/1
  StrWhSnis_state/1(IMU_BUS) -> StrWhSnis_BUS/1  "SWAS"
  CANReceive3/1 -> StrWhSnis_state/Trigger
  CANReceive3/4 -> StrWhSnis_state/3(Msg)
  CANReceive3/3 -> StrWhSnis_state/2(ID)

== system VehCtrlMdel240912_2018b/Input/key ==
  function : TriggerPort  TriggerType=function-call  VariantControl=(inherit)
  Bus Creator : BusCreator  Inputs=3
  Logical Operator : Logic  Operator=NOT  AllPortsSameDT=off  OutDataTypeStr=boolean
  MeaModule : ec5744lib/RapidECU_U3/07Calibration/MeaModule  signal=ignition
      settings: SourceProductName=ECUCoder for MPC5744
  SwitchInput : ec5744lib/RapidECU_U3/01BasicInput/SwitchInput  channel=6:I_SW01_L  sampletime=-1
      settings: SourceProductName=ECUCoder for MPC5744
  SwitchInput1 : ec5744lib/RapidECU_U3/01BasicInput/SwitchInput  channel=7:I_SW02_L  sampletime=-1
      settings: SourceProductName=ECUCoder for MPC5744
  SwitchInput2 : ec5744lib/RapidECU_U3/01BasicInput/SwitchInput  channel=8:I_SW03_L  sampletime=-1
      settings: SourceProductName=ECUCoder for MPC5744
  key : Outport  VectorParamsAs1DForOutWhenUnconnected=off
  wires:
  SwitchInput/1 -> Logical Operator/1  "Drive_ready"
  SwitchInput1/1 -> Bus Creator/1  "AMKCLDCON"
  Bus Creator/1 -> key/1
  MeaModule/1 -> Bus Creator/2  "ignition"
  Logical Operator/1 -> MeaModule/1
  SwitchInput2/1 -> Bus Creator/3  "HVCUTOFF"

== system VehCtrlMdel240912_2018b/Input_Processing/Function-Call Subsystem ==
  INPUT_BUS : Inport
  function : TriggerPort  TriggerType=function-call  VariantControl=Variant
  AccBrkPedal : Subsystem
  Bus Selector : BusSelector  OutputSignals=IMU,AccBrk_BUS,SWAS,ABS_BUS,AMKMCUtoVCU_BUS
  Bus Creator : BusCreator  Inputs=5
  IMU : Subsystem
  SWAS : Subsystem
  WhlSpdii_mps : Subsystem
  Out1 : Outport  VectorParamsAs1DForOutWhenUnconnected=off
  wires:
  INPUT_BUS/1 -> [BUS], Bus Selector/1  "BUS"
  Bus Selector/1 -> IMU/1(IMU)  "<IMU>"
  Bus Selector/2 -> AccBrkPedal/1(AccBrk_BUS)  "<AccBrk_BUS>"
  Bus Selector/3 -> SWAS/1(SWAS)  "<SWAS>"
  Bus Selector/4 -> WhlSpdii_mps/1(IMU)  "<ABS_BUS>"
  Bus Selector/5 -> WhlSpdii_mps/2(In2)  "<AMKMCUtoVCU_BUS>"
  IMU/1(IMU_BUS) -> Bus Creator/1  "IMU_Processing"
  AccBrkPedal/1(AccBrk) -> Bus Creator/2  "AccBrkPedal_Processing"
  SWAS/1(StrWhlAng&V) -> Bus Creator/3  "SWAS_Processing"
  WhlSpdii_mps/1(WhlSpdii_mps) -> Bus Creator/4  "WhlSpdii_mps"
  Bus Creator/1 -> Out1/1
  [BUS] -> Bus Creator/5

== system VehCtrlMdel240912_2018b/Input_Processing/Subsystem ==
  note: 和实车相反
  note: 信号的滤波去噪应该在其他模块完成
  OutPutBus : Inport
  function : TriggerPort  TriggerType=function-call  VariantControl=(inherit)
  Bus Selector : BusSelector  OutputSignals=WhlSpdii_mps.WhlSpdFL,WhlSpdii_mps.WhlSpdFR,WhlSpdii_mps.WhlSpdRL_mps,WhlSpdii_mps.WhlSpdRR_mps,IMU_Processing.IMU_Yaw_Value,SWAS_Processing.FLWhlStrAng,SWAS_Processing.FRWhlStrAng,IMU_Processing.IMU_Ax_Valid,BUS.IMU.IMU_Ax_Valid,AccBrkPedal_Processing.Acc_POS
  Cast To Double{,1..7} (8 alike) : DataTypeConversion  OutDataTypeStr=single
  From : From  Commented=on  GotoTag=IMU_Aa_mpss
  Gain5 : Gain  Gain=10
  "IntglJudgment " : Subsystem
  Unit Delay : UnitDelay  SampleTime=-1  HasFrameUpgradeWarning=on
  Unit Delay1 : UnitDelay  SampleTime=-1  HasFrameUpgradeWarning=on
  WhlSlpageJudgment : Subsystem
  WhlSpdSelect : Subsystem
  坐标系转换 : Subsystem
  VehVxEst_mps : Outport
  Vxii_mps : Outport  Port=2
  wires:
  Bus Selector/10 -> "IntglJudgment "/8(Acc_POS)  "<Acc_POS>"
  WhlSlpageJudgment/1(WhlSlipFLValid_flag) -> "IntglJudgment "/1(WhlSlipFL_flag), WhlSpdSelect/1(WhlSlipFL_flag)
  WhlSlpageJudgment/5(WhlSpdMax_mps) -> [WhlSpdMax_mps]
  "IntglJudgment "/2(IMUVehSpdEstiExit) -> WhlSpdSelect/8(IMUVehSpdEstiExit)
  WhlSlpageJudgment/2(WhlSlipFRValid_flag) -> "IntglJudgment "/2(WhlSlipFR_flag), WhlSpdSelect/2(WhlSlipFR_flag)
  Bus Selector/8 -> Gain5/1  "<IMU_Ax_Valid>"
  "IntglJudgment "/1(VxIMU_est) -> WhlSpdSelect/7(VxIMU_est)
  WhlSlpageJudgment/3(WhlSlipRLValid_flag) -> "IntglJudgment "/3(WhlSlipRL_flag), WhlSpdSelect/3(WhlSlipRL_flag)
  Cast To Double1/1 -> 坐标系转换/1(WhlSpdFL_mps)
  [IMU_Aa_mpss] -> WhlSpdSelect/6(IMU_Ax_mpss)
  Unit Delay1/1 -> "IntglJudgment "/7(FFVehVxEst_mps)
  [Vxii_mps] -> Vxii_mps/1, WhlSpdSelect/5(Vxii_mps)
  Cast To Double7/1 -> 坐标系转换/7(WhlStrAngR_deg)  "WhlStrAngR_deg"
  Bus Selector/4 -> Cast To Double4/1  "<WhlSpdRR_mps>"
  Cast To Double4/1 -> 坐标系转换/4(WhlSpdRR_mps)
  Cast To Double/1 -> [IMU_Aa_mpss], WhlSlpageJudgment/3(IMU_Aa_mpss)
  Cast To Double2/1 -> 坐标系转换/2(WhlSpdFR_mps)
  [VehVxEst_mps] -> Unit Delay/1
  WhlSlpageJudgment/4(WhlSlipRRValid_flag) -> WhlSpdSelect/4(WhlSlipRR_flag), "IntglJudgment "/4(WhlSlipRR_flag)
  WhlSpdSelect/1(VehVxEst1_mps) -> VehVxEst_mps/1, [VehVxEst_mps]  "VehVxEst_mps"
  坐标系转换/1(Vxii_mps) -> [Vxii_mps], WhlSlpageJudgment/1(Vxii_mps)  "Vxii_mps"
  Cast To Double5/1 -> 坐标系转换/5(IMU_YawRate_dps)  "IMU_YawRate_dps"
  Cast To Double3/1 -> 坐标系转换/3(WhlSpdRL_mps)
  [VehVxEst_mps] -> Unit Delay1/1
  坐标系转换/2(IMU_YawRate_dps1) -> WhlSlpageJudgment/2(IMU_YawRate_dps)  "IMU_YawRate_dps"
  Bus Selector/3 -> Cast To Double3/1  "<WhlSpdRL_mps>"
  [WhlSpdMax_mps] -> "IntglJudgment "/9(WhlSpdMax_mps)
  Bus Selector/1 -> Cast To Double1/1  "<WhlSpdFL>"
  Bus Selector/2 -> Cast To Double2/1  "<WhlSpdFR>"
  Unit Delay/1 -> WhlSlpageJudgment/4(VehSpdEstiZ1_mps)
  Cast To Double6/1 -> 坐标系转换/6(WhlStrAngL_deg)  "WhlStrAngL_deg"
  Gain5/1 -> Cast To Double/1  "IMU_Ax_mpss"
  Bus Selector/5 -> Cast To Double5/1  "<IMU_Yaw_Value>"
  Bus Selector/6 -> Cast To Double6/1  "<FLWhlStrAng>"
  Bus Selector/7 -> Cast To Double7/1  "<FRWhlStrAng>"
  WhlSpdSelect/2(AccEst_mpss) -> [AccEst_mpss]
  [AccEst_mpss] -> "IntglJudgment "/6(IMU_Ax_mpss)
  OutPutBus/1 -> [OUTPUTBUS], Bus Selector/1
  Bus Selector/9 -> "IntglJudgment "/5(Ax_Valid)  "<IMU_Ax_Valid>"
  [OUTPUTBUS] -> WhlSlpageJudgment/5(In5)

== system VehCtrlMdel240912_2018b/OUTPUT/Beeper ==
  Beeper_state : Inport
  function : TriggerPort  TriggerType=function-call  VariantControl=(inherit)
  MeaModule : ec5744lib/RapidECU_U3/07Calibration/MeaModule  signal=beeper_state
      settings: SourceProductName=ECUCoder for MPC5744
  PowerDriverSwitch(HS) : ec5744lib/RapidECU_U3/02PowerDriverSwitch/PowerDriverSwitch(HS)  channel=117:O_SW14_HS1A  sampletime=-1
      settings: SourceProductName=ECUCoder for MPC5744
  wires:
  Beeper_state/1 -> MeaModule/1
  MeaModule/1 -> PowerDriverSwitch(HS)/1

== system VehCtrlMdel240912_2018b/OUTPUT/VCU2AMKMCUFL ==
  MCFL_TargetTorque : Inport
  In2 : Inport  Port=2
  function : TriggerPort  TriggerType=function-call  VariantControl=(inherit)
  Bus Selector : BusSelector  OutputSignals=MCFL_DCOn_setpoints,MCFL_DCEnable,errorReset,MCFL_InverterOn
  CAN Pack1 : canmsglib/CAN Pack  CANdbFile=C:\Users\12045\Desktop\DBC\DRe20_dbc_v1.16\DRe20_dbc_v1.16_CAN2.dbc  MsgList=(none)  MsgName=MCFL_SetPoints  MsgIDType=Standard (11-bit identifier)  MsgIdentifier=386  MsgLength=8  Remote=off  ApplyMinMax=off  BusOutput=off  SignalInfo={'MCFL_TargetTorque','16','16','LE','signed','Standard','0','0.0098','0','-Inf','Inf';'MCFL_TorqueLimitN','48','16','LE','signed','Standard','0','0.0098','0','-Inf','Inf';'MCFL_TorqueLimitP','32','16','LE','signed','Standard','0','0.0098','0','-Inf','Inf';'MCFL_cDCOn','9','1','LE','unsigned','Standard','0','1','0','0','1';'MCFL_cEnable','10','1','LE','unsigned','Standard','0','1','0','0','1';'MCFL_cErrorReset','11','1','LE','unsigned','Standard','0','1','0','0','1';'MCFL_cInverterOn','8','1','LE','unsigned','Standard','0','1','0','0','1';'MCFL_cReserve1','0','8','LE','unsigned','Standard','0','1','0','-Inf','Inf';'MCFL_cReserve2','12','4','LE','unsigned','Standard','0','1','0','-Inf','Inf'}
      settings: SourceProductName=Vehicle Network Toolbox  SourceProductBaseCode=VN  DataFormat=CANdb specified signals
  CANPackMessage : ec5744lib/RapidECU_U3/04CANCommunication/CANPackMessage  datalength=8  sampletime=-1
      settings: SourceProductName=ECUCoder for MPC5744
  CANTransmit : ec5744lib/RapidECU_U3/04CANCommunication/CANTransmit  canmodule=1  canbuffer=8  canmessageid=386  canmessagetype=Extended(29-bit ID)  datalength=8  sampletime=-1
      settings: SourceProductName=ECUCoder for MPC5744
  Constant : Constant  Value=1000
  Constant1 : Constant  Value=0
  Ground1 : Ground
  Ground2 : Ground
  Terminator3 : Terminator
  wires:
  CANPackMessage/1 -> CANTransmit/1
  CAN Pack1/1 -> CANPackMessage/1
  CANTransmit/1 -> Terminator3/1
  MCFL_TargetTorque/1 -> CAN Pack1/1  "MCFL_TargetTorque"
  Constant1/1 -> CAN Pack1/2  "MCFL_TorqueLimitN"
  Bus Selector/1 -> CAN Pack1/4  "<MCFL_DCOn_setpoints>"
  Constant/1 -> CAN Pack1/3  "MCFL_TorqueLimitP"
  Ground1/1 -> CAN Pack1/8  "MCFL_cReserve1"
  Bus Selector/4 -> CAN Pack1/7  "<MCFL_InverterOn>"
  Bus Selector/2 -> CAN Pack1/5  "<MCFL_DCEnable>"
  Ground2/1 -> CAN Pack1/9  "MCFL_cReserve2"
  In2/1 -> Bus Selector/1
  Bus Selector/3 -> CAN Pack1/6  "<errorReset>"

== system VehCtrlMdel240912_2018b/OUTPUT/VCU2AMKMCUFR ==
  <BUS> : Inport
  In1 : Inport  Port=2
  function : TriggerPort  TriggerType=function-call  VariantControl=(inherit)
  Bus Selector : BusSelector  OutputSignals=MCFL_DCOn_setpoints,MCFL_DCEnable,errorReset,MCFL_InverterOn
  CAN Pack1 : canmsglib/CAN Pack  CANdbFile=C:\Users\12045\Desktop\DBC\DRe20_dbc_v1.16\DRe20_dbc_v1.16_CAN2.dbc  MsgList=(none)  MsgName=MCFR_SetPoints  MsgIDType=Standard (11-bit identifier)  MsgIdentifier=387  MsgLength=8  Remote=off  ApplyMinMax=off  BusOutput=off  SignalInfo={'MCFR_TargetTorque','16','16','LE','signed','Standard','0','0.0098','0','-Inf','Inf';'MCFR_TorqueLimitN','48','16','LE','signed','Standard','0','0.0098','0','-Inf','Inf';'MCFR_TorqueLimitP','32','16','LE','signed','Standard','0','0.0098','0','-Inf','Inf';'MCFR_cDCOn','9','1','LE','unsigned','Standard','0','1','0','0','1';'MCFR_cEnable','10','1','LE','unsigned','Standard','0','1','0','0','1';'MCFR_cErrorReset','11','1','LE','unsigned','Standard','0','1','0','0','1';'MCFR_cInverterOn','8','1','LE','unsigned','Standard','0','1','0','0','1';'MCFR_cReserve1','0','8','LE','unsigned','Standard','0','1','0','-Inf','Inf';'MCFR_cReserve2','12','4','LE','unsigned','Standard','0','1','0','-Inf','Inf'}
      settings: SourceProductName=Vehicle Network Toolbox  SourceProductBaseCode=VN  DataFormat=CANdb specified signals
  CANPackMessage : ec5744lib/RapidECU_U3/04CANCommunication/CANPackMessage  datalength=8  sampletime=-1
      settings: SourceProductName=ECUCoder for MPC5744
  CANTransmit : ec5744lib/RapidECU_U3/04CANCommunication/CANTransmit  canmodule=1  canbuffer=8  canmessageid=146927393  canmessagetype=Extended(29-bit ID)  datalength=8  sampletime=-1
      settings: SourceProductName=ECUCoder for MPC5744
  Constant : Constant  Value=0
  Constant1 : Constant  Value=1000
  Ground : Ground
  Ground1 : Ground
  Terminator3 : Terminator
  wires:
  Ground1/1 -> CAN Pack1/9  "MCFR_cReserve2"
  Bus Selector/2 -> CAN Pack1/5  "<MCFL_DCEnable>"
  Bus Selector/3 -> CAN Pack1/6  "<errorReset>"
  Bus Selector/4 -> CAN Pack1/7  "<MCFL_InverterOn>"
  Ground/1 -> CAN Pack1/8  "MCFR_cReserve1"
  Constant1/1 -> CAN Pack1/3  "MCFR_TorqueLimitP"
  Bus Selector/1 -> CAN Pack1/4  "<MCFL_DCOn_setpoints>"
  Constant/1 -> CAN Pack1/2  "MCFR_TorqueLimitN"
  CANTransmit/1 -> Terminator3/1
  CAN Pack1/1 -> CANPackMessage/1
  CANPackMessage/1 -> CANTransmit/1
  In1/1 -> CAN Pack1/1
  <BUS>/1 -> Bus Selector/1
